simulink model "opg5"  (R2018b)
settings: Solver=VariableStepAuto  StartTime=0.0  StopTime=10.0  RelTol=1e-3
values from neighbouring files (symbols this model uses):
  H1den = fliplr(H1den)    [opg5.m]    (also in opg5_matlab.m = sos(1:1,4:6))
  H1num = fliplr(H1num)    [opg5.m]    (also in opg5_matlab.m = sos(1:1,1:3))
  H2num = fliplr(H2num)    [opg5.m]    (also in opg5_matlab.m = sos(2:2,1:3))
  H3den = fliplr(H3den)    [opg5.m]    (also in opg5_matlab.m = sos(3:3,4:6))
  H3num = fliplr(H3num)    [opg5.m]    (also in opg5_matlab.m = sos(3:3,1:3))
settings Model: Creator=kasper  LastModifiedBy=kasper

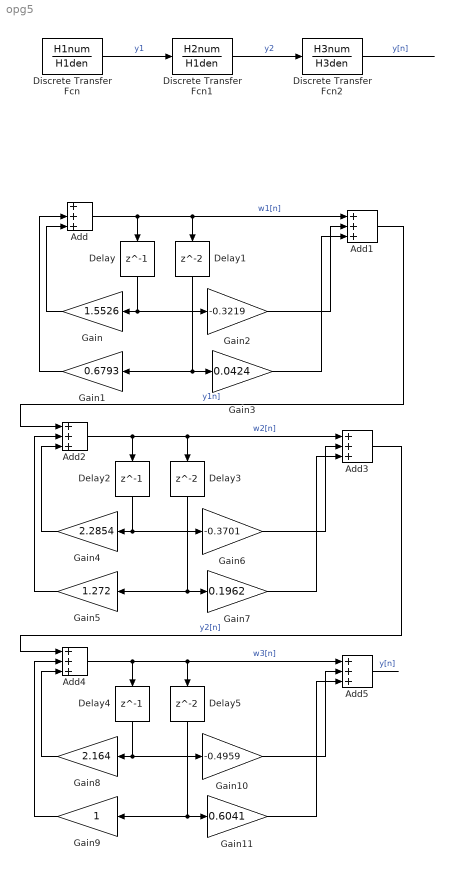
== system opg5 ==
  Add{,1..5} (6 alike) : Sum  Inputs=+++
  Delay : Delay  DelayLength=1
  Delay1 : Delay
  Delay2 : Delay  DelayLength=1
  Delay3 : Delay
  Delay4 : Delay  DelayLength=1
  Delay5 : Delay
  Discrete Transfer Fcn : DiscreteTransferFcn  Numerator=H1num  Denominator=H1den
  Discrete Transfer Fcn1 : DiscreteTransferFcn  Numerator=H2num  Denominator=H1den
  Discrete Transfer Fcn2 : DiscreteTransferFcn  Numerator=H3num  Denominator=H3den
  Gain : Gain  Gain=1.5526
  Gain1 : Gain  Gain=0.6793
  Gain10 : Gain  Gain=-0.4959
  Gain11 : Gain  Gain=0.6041
  Gain2 : Gain  Gain=-0.3219
  Gain3 : Gain  Gain=0.0424
  Gain4 : Gain  Gain=2.2854
  Gain5 : Gain  Gain=1.272
  Gain6 : Gain  Gain=-0.3701
  Gain7 : Gain  Gain=0.1962
  Gain8 : Gain  Gain=2.164
  Gain9 : Gain
  wires:
  Discrete Transfer Fcn1/1 -> Discrete Transfer Fcn2/1  "y2"
  Discrete Transfer Fcn/1 -> Discrete Transfer Fcn1/1  "y1"
  ? -> Discrete Transfer Fcn/1  "x[n]"
  Discrete Transfer Fcn2/1 -> ?  "y[n]"
  Delay/1 -> Gain/1, Gain2/1
  Delay1/1 -> Gain1/1, Gain3/1
  Gain/1 -> Add/3
  Gain1/1 -> Add/2
  Add/1 -> Delay/1, Add1/1, Delay1/1  "w1[n]"
  ? -> Add/1  "x[n]"
  Gain2/1 -> Add1/2
  Gain3/1 -> Add1/3
  Add2/1 -> Delay2/1, Add3/1, Delay3/1  "w2[n]"
  Gain4/1 -> Add2/3
  Gain6/1 -> Add3/2
  Delay2/1 -> Gain4/1, Gain6/1
  Gain7/1 -> Add3/3
  Add1/1 -> Add2/1  "y1n]"
  Delay3/1 -> Gain5/1, Gain7/1
  Gain5/1 -> Add2/2
  Add4/1 -> Delay4/1, Add5/1, Delay5/1  "w3[n]"
  Gain8/1 -> Add4/3
  Gain10/1 -> Add5/2
  Delay4/1 -> Gain8/1, Gain10/1
  Gain11/1 -> Add5/3
  Delay5/1 -> Gain9/1, Gain11/1
  Gain9/1 -> Add4/2
  Add3/1 -> Add4/1  "y2[n]"
  Add5/1 -> ?  "y[n]"
